simulink model "CubeX_LQR_3D"  (R2017b)
settings: Solver=FixedStepDiscrete  StartTime=0.0  StopTime=inf  FixedStep=Ts.base  RelTol=1e-3
PreLoadFcn:
  | waijung.modelPreload; % Required for working with Waijung Blockset. Do not remove.
InitFcn:
  | cubeparameters
  | LQR_3d
undefined symbols (not defined in the file or in its folder): deg_, g, HSEOSC, imu, K_lqr_3D, Link, LQFP176, motor, ST, STM32F417IG, Ts
libraries: simulink x29, stm32f4_i2c_lib x8, stm32f4_io_lib x7, stm32f4_adc_lib x3, stm32f4_device_config_lib x1, BC_USB x1
(part 1 of 3)
CloseFcn:
  | waijung.modelClose; % Required for working with Waijung Blockset. Do not remove.
settings Model: Creator=Hi  LastModifiedBy=Love
settings DataIOCC: LimitDataPoints=on  SaveFormat=Array
settings OptimizationCC: LifeSpan=1
settings DebuggingCC: AllowSymbolicDim=off  SFUnexpectedBacktrackingDiag=warning  SFNoUnconditionalDefaultTransitionDiag=warning  SFExecutionAtInitializationDiag=none
settings HardwareCC: ProdBitPerPointer=32  ProdBitPerSizeT=32  ProdBitPerPtrDiffT=32  ProdLargestAtomicFloat=None  ProdIntDivRoundTo=Undefined  ProdWordSize=32  ProdHWDeviceType=ARM Compatible->Cortex - M4  TargetEndianess=LittleEndian  TargetHWDeviceType=ARM Compatible->Cortex - M4
settings ModelReferenceCC: PropagateSignalLabelsOutOfModel=off
settings SFSimCC: MATLABDynamicMemAlloc=off
settings RTWCC: SystemTargetFile=stm32f4.tlc  GenerateMakefile=off  TemplateMakefile=ert_default_tmf  Description=STM32F4 Target
settings CodeAppCC: ForceParamTrailComments=on  IgnoreCustomStorageClasses=off  OperatorAnnotations=on  SimulinkDataObjDesc=on  InsertBlockDesc=on  StateflowObjectComments=on  MATLABSourceComments=on
settings STFCustomTargetCC: ModelReferenceCompliant=off  CombineOutputUpdateFcns=on  ERTCustomFileBanners=on  SupportContinuousTime=off  SupportNonInlinedSFcns=off  RemoveResetFunc=on  MATLABClassNameForMDSCustomization=Simulink.SoftwareTarget.ERTCustomization  GRTInterface=off  SystemTargetFile=stm32f4.tlc
settings ERTTargetCC: MultiwordLength=2048  ModelReferenceCompliant=off  ParMdlRefBuildCompliant=off  CompOptLevelCompliant=off  ConcurrentExecutionCompliant=off  ModelStepFunctionPrototypeControlCompliant=off  CPPClassGenCompliant=off  UseToolchainInfoCompliant=off  ERTSrcFileBannerTemplate=stm32f4_code_template.cgt  ERTHdrFileBannerTemplate=stm32f4_code_template.cgt  ERTDataSrcFileTemplate=stm32f4_code_template.cgt  ERTDataHdrFileTemplate=stm32f4_code_template.cgt  ERTCustomFileTemplate=stm32f4_file_process.tlc  ConvertIfToSwitch=off  SuppressUnreachableDefaultCases=off
settings ConfigComp: CovMetricSettings=dw  CovHtmlReporting=on  CovSaveCumulativeToWorkspaceVar=on  CovSaveSingleToWorkspaceVar=on  CovExternalEMLEnable=off

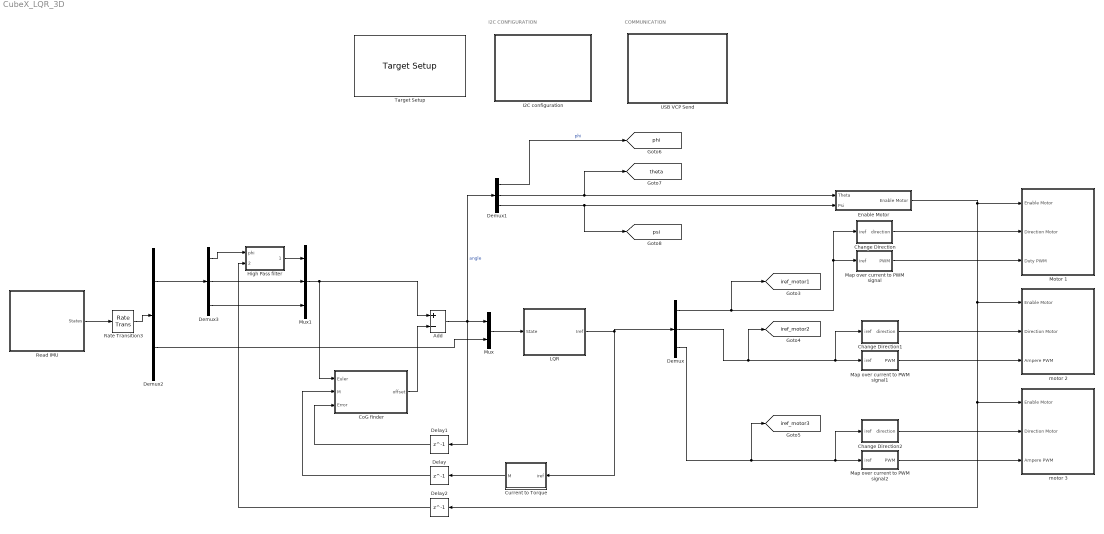
== system CubeX_LQR_3D ==
  note: COMMUNICATION
  note: I2C CONFIGURATION
  Add : Sum  Inputs=+-
  Change Direction : Subsystem
  Change Direction1 : Subsystem
  Change Direction2 : Subsystem
  CoG finder : Subsystem
  Current to Torque : Subsystem
  Delay : Delay  DelayLength=1  InitialCondition=[0 0 0]'
  Delay1 : Delay  DelayLength=1  InitialCondition=[0 0 0]'
  Delay2 : Delay  DelayLength=1  InitialCondition=0
  Demux : Demux  Outputs=3
  Demux1 : Demux  Outputs=3
  Demux2 : Demux  Outputs=2
  Demux3 : Demux  Outputs=3
  Enable Motor : Subsystem  SystemSampleTime=Ts.controller
  High Pass filter : MATLAB Function  TreatAsAtomicUnit=on
  I2C configuration : Subsystem
  LQR : Subsystem
  Map over current to PWM signal : Subsystem
  Map over current to PWM signal1 : Subsystem
  Map over current to PWM signal2 : Subsystem
  Motor 1 : Subsystem
  Mux : Mux  Inputs=2
  Mux1 : Mux  Inputs=3
  Rate Transition3 : RateTransition  OutPortSampleTime=Ts.controller
  Read IMU : Subsystem
  Target Setup : stm32f4_device_config_lib/Target Setup  Priority=100  compiler=GNU ARM  previous_compiler=GNU ARM  mcu=STM32F417IG (LQFP176)  mcustr=STM32F417IG  clockconfig=HSEOSC-8MHz  system_stm32f4xx_c_path=C:\waijung15_04a\targets\stm32f4_target\stm32f4\utils\STM32F4xx_AN3988_V1.0.1\stm32f4_default\hseosc8mhz  showmemoryconfiguration=off  stacksize=0x400  heapsize=0x200  enableautocompiledownload=on  fullchiperase=off  programmerinterface=ST-Link  editctrlstr=on  compilercontrolstr=$(patsubst %, -I%, .) -mcpu=cortex-m4 -mthumb -mthumb-interwork -mfloat-abi=hard -mfpu=fpv4-sp-d16 -ffast-math -Wall -Wextra -Ofast  assemblercontrolstr=$(patsubst %, -I%, .) -mcpu=cortex-m4 -mthumb -mthumb-interwork -mfloat-abi=hard -mfpu=fpv4-sp-d16 -ffast-math -Wall -Wextra -Ofast -Wa,-amhls=$(<:.s=.lst) -D__STACK_SIZE=$(STACK_SIZE) -D__HEAP_SIZE=$(HEAP_SIZE)  linkercontrolstr=-T$(LD_SCRIPT) -g -Wl,-Map=$(MAP),--cref,--no-warn-mismatch -mcpu=cortex-m4 -mthumb -mthumb-interwork -mfloat-abi=hard -mfpu=fpv4-sp-d16  runafterdownload=on  execprofile=None  profileruart=1  profilerbaud=115200  profilertxpin=D8  profilerinitstr=0.002,168000000,336000,115200,0  manualsetsampletime=on  sampletime=0.002  blockid=TargetSetup  systickreloadvalue=336000  hseval=8000000  lastprofileruart=1  hclk=168000000  flashorigin=0x8000000  flashlength=1M  ramorigin=0x20000000  ramlength=112k  useextram=off
  USB VCP Send : Subsystem
  motor 2 : Subsystem
  "motor 3 " : Subsystem
  tag scope: iref_motor1=global, iref_motor2=global, iref_motor3=global, phi=global, psi=global, theta=global
  wires:
  Map over current to PWM signal/1(PWM) -> Motor 1/3(Duty PWM)
  Change Direction/1(direction) -> Motor 1/2("Direction Motor ")
  Enable Motor/1(Enable Motor) -> motor 2/1(Enable Motor), "motor 3 "/1(Enable Motor), Delay2/1, Motor 1/1(Enable Motor)
  CoG finder/1(offset) -> Add/2
  Change Direction1/1(direction) -> motor 2/2("Direction Motor ")
  Change Direction2/1(direction) -> "motor 3 "/2("Direction Motor ")
  Map over current to PWM signal2/1(PWM) -> "motor 3 "/3(Ampere PWM)
  Map over current to PWM signal1/1(PWM) -> motor 2/3(Ampere PWM)
  Add/1 -> Demux1/1, Delay1/1, Mux/1  "angle"
  Mux/1 -> LQR/1(State)
  LQR/1(Iref) -> Current to Torque/1(iref), Demux/1
  Read IMU/1(States) -> Rate Transition3/1
  Rate Transition3/1 -> Demux2/1
  Demux2/2 -> Mux/2
  Delay/1 -> CoG finder/2(M)
  Delay1/1 -> CoG finder/3(Error)
  Demux2/1 -> Demux3/1
  Demux3/1 -> High Pass filter/1(phi)
  High Pass filter/1(phi_zero) -> Mux1/1
  Demux3/2 -> Mux1/2
  Demux3/3 -> Mux1/3
  Mux1/1 -> CoG finder/1(Euler), Add/1
  Delay2/1 -> High Pass filter/2(motor_enable)
  Demux1/2 -> [theta], Enable Motor/1(Theta)
  Demux1/3 -> [psi], Enable Motor/2(Psi)
  Demux1/1 -> [phi]  "phi"
  Demux/2 -> Change Direction1/1(iref), Map over current to PWM signal1/1(iref), [iref_motor2]
  Demux/3 -> Change Direction2/1(iref), Map over current to PWM signal2/1(iref), [iref_motor3]
  Demux/1 -> [iref_motor1], Change Direction/1(iref), Map over current to PWM signal/1(iref)
  Current to Torque/1(M) -> Delay/1

== system CubeX_LQR_3D/Change Direction ==
  iref : Inport
  Compare To Zero : simulink/Logic and Bit Operations/Compare To Zero  relop=>=  OutDataTypeStr=boolean
  direction : Outport
  wires:
  iref/1 -> Compare To Zero/1
  Compare To Zero/1 -> direction/1

== system CubeX_LQR_3D/Change Direction1 ==
  iref : Inport
  Compare To Zero : simulink/Logic and Bit Operations/Compare To Zero  relop=>=  OutDataTypeStr=boolean
  direction : Outport
  wires:
  iref/1 -> Compare To Zero/1
  Compare To Zero/1 -> direction/1

== system CubeX_LQR_3D/Change Direction2 ==
  iref : Inport
  Compare To Zero : simulink/Logic and Bit Operations/Compare To Zero  relop=>=  OutDataTypeStr=boolean
  direction : Outport
  wires:
  iref/1 -> Compare To Zero/1
  Compare To Zero/1 -> direction/1

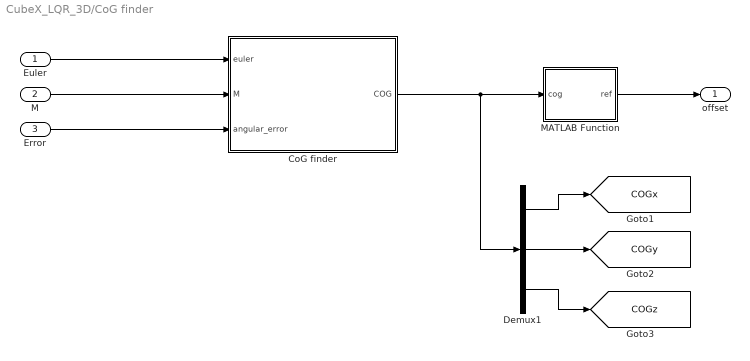
== system CubeX_LQR_3D/CoG finder ==
  Euler : Inport
  M : Inport  Port=2
  Error : Inport  Port=3
  CoG finder : MATLAB Function  TreatAsAtomicUnit=on
  Demux1 : Demux  Outputs=3
  MATLAB Function : MATLAB Function  TreatAsAtomicUnit=on
  offset : Outport
  tag scope: COGx=global, COGy=global, COGz=global
  wires:
  CoG finder/1(COG) -> Demux1/1, MATLAB Function/1(cog)
  MATLAB Function/1(ref) -> offset/1
  Demux1/2 -> [COGy]
  Demux1/3 -> [COGz]
  Demux1/1 -> [COGx]
  Euler/1 -> CoG finder/1(euler)
  Error/1 -> CoG finder/3(angular_error)
  M/1 -> CoG finder/2(M)

== system CubeX_LQR_3D/Current to Torque ==
  iref : Inport
  "Gain " : Gain  Gain=motor.kt
  M : Outport
  wires:
  iref/1 -> "Gain "/1
  "Gain "/1 -> M/1

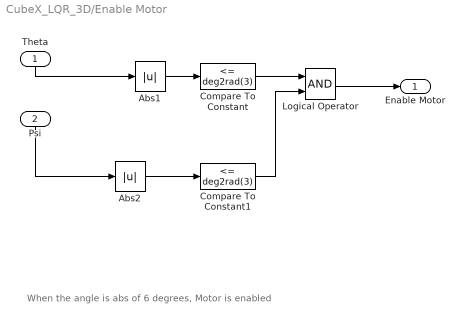
== system CubeX_LQR_3D/Enable Motor ==
  note: When the angle is abs of 6 degrees, Motor is enabled
  Theta : Inport
  Psi : Inport  Port=2
  Abs1 : Abs
  Abs2 : Abs
  Compare To Constant : simulink/Logic and Bit Operations/Compare To Constant  relop=<=  const=deg2rad(3)  OutDataTypeStr=boolean
  Compare To Constant1 : simulink/Logic and Bit Operations/Compare To Constant  relop=<=  const=deg2rad(3)  OutDataTypeStr=boolean
  Logical Operator : Logic  AllPortsSameDT=off  OutDataTypeStr=boolean
  Enable Motor : Outport
  wires:
  Abs1/1 -> Compare To Constant/1
  Theta/1 -> Abs1/1
  Psi/1 -> Abs2/1
  Abs2/1 -> Compare To Constant1/1
  Compare To Constant/1 -> Logical Operator/1
  Compare To Constant1/1 -> Logical Operator/2
  Logical Operator/1 -> Enable Motor/1

== system CubeX_LQR_3D/I2C configuration ==
  I2C Master Setup1 : S-Function  FunctionName=stm32f4_i2c  Parameters=configuration,module,transfer,clkspeed,timeout,sdapin,sclpin,writecount,readcount,inputtypearray,outputtypearray,confstr,sampletime,sampletimestr,blockid  SFunctionDeploymentMode=off  EnableBusSupport=off  mask(stm32f4_i2c){configuration=Setup, module=3, lastmodule=3, transfer=Blocking, dutycycle=TLow/THigh = 2, clkspeed=400, timeout=25, writecount=0, readcount=0, sdapin=C9, sclpin=A8, waitwritetime=0, inputtypearray=[0], outputtypearray=[0], confstr=["C","9","A","8","1","3","4","2","I2C_DutyCycle_2","0","off"], sampletime=-1, sampletimestr=0.002, blockid=I2CconfigurationI2CMasterSetup1}
      mask prompts: module "I2C Module"; lastmodule "Last module"; transfer "Transfer mode"; dutycycle "Duty cycle in fast mode"; clkspeed "Clock speed (kHz)"; timeout "Timeout (ms)"; writecount "Bytes write count"; readcount "Bytes read count"; sdapin "SDA pin"; sclpin "SCL pin"; waitwritetime "Wait write time (ms), default is 0"; inputtypearray "Input type array"; outputtypearray "Output type array"; confstr "Configuration string"; sampletime "Sample time (sec)"; sampletimestr "Compiled sample time (sec) in string"
      mask init:
      | stm32f4_i2c_callback('init');
      mask Help: web(fullfile(waijungdocroot,'stm32f4_i2c_setup.htm'), '-browser')
      mask TypeOptions configuration: Setup | Transaction
      mask Callback configuration: stm32f4_i2c_callback('configuration');
      mask TypeOptions module: 1 | 2 | 3
      mask Callback module: stm32f4_i2c_callback('module');
      mask TypeOptions transfer: Blocking | Non-blocking
      mask TypeOptions dutycycle: TLow/THigh = 16/9 | TLow/THigh = 2
      mask Callback dutycycle: stm32f4_i2c_callback('dutycycle');
      mask Callback writecount: stm32f4_i2c_callback('writecount');
      mask Callback readcount: stm32f4_i2c_callback('readcount');
      mask TypeOptions sdapin: - | C9
      mask Callback sdapin: stm32f4_i2c_callback('sdapin');
      mask TypeOptions sclpin: - | A8
      mask Callback sclpin: stm32f4_i2c_callback('sclpin');
      mask Callback confstr: stm32f4_i2c_callback('confstr');
      mask Callback sampletime: stm32f4_i2c_callback('sampletime');
      mask Callback sampletimestr: stm32f4_i2c_callback('sampletimestr');
      mask Callback blockid: stm32f4_i2c_callback('blockid');
      mask Display: text(0.5, 0.5, 'Module: I2C3\nClock: 400kHz\nSDA/SCL Pin: C9/A8','ver','middle','hor','center');
  I2C Master Setup2 : S-Function  FunctionName=stm32f4_i2c  Parameters=configuration,module,transfer,clkspeed,timeout,sdapin,sclpin,writecount,readcount,inputtypearray,outputtypearray,confstr,sampletime,sampletimestr,blockid  SFunctionDeploymentMode=off  EnableBusSupport=off  mask(stm32f4_i2c){configuration=Setup, module=1, lastmodule=1, transfer=Blocking, dutycycle=TLow/THigh = 2, clkspeed=400, timeout=25, writecount=0, readcount=0, sdapin=B9, sclpin=B6, waitwritetime=0, inputtypearray=[0], outputtypearray=[0], confstr=["B","9","B","6","1","1","6","0","I2C_DutyCycle_2","0","off"], sampletime=-1, sampletimestr=0.002, blockid=I2CconfigurationI2CMasterSetup2}
      mask prompts: module "I2C Module"; lastmodule "Last module"; transfer "Transfer mode"; dutycycle "Duty cycle in fast mode"; clkspeed "Clock speed (kHz)"; timeout "Timeout (ms)"; writecount "Bytes write count"; readcount "Bytes read count"; sdapin "SDA pin"; sclpin "SCL pin"; waitwritetime "Wait write time (ms), default is 0"; inputtypearray "Input type array"; outputtypearray "Output type array"; confstr "Configuration string"; sampletime "Sample time (sec)"; sampletimestr "Compiled sample time (sec) in string"
      mask init:
      | stm32f4_i2c_callback('init');
      mask Help: web(fullfile(waijungdocroot,'stm32f4_i2c_setup.htm'), '-browser')
      mask TypeOptions configuration: Setup | Transaction
      mask Callback configuration: stm32f4_i2c_callback('configuration');
      mask TypeOptions module: 1 | 2 | 3
      mask Callback module: stm32f4_i2c_callback('module');
      mask TypeOptions transfer: Blocking | Non-blocking
      mask TypeOptions dutycycle: TLow/THigh = 16/9 | TLow/THigh = 2
      mask Callback dutycycle: stm32f4_i2c_callback('dutycycle');
      mask Callback writecount: stm32f4_i2c_callback('writecount');
      mask Callback readcount: stm32f4_i2c_callback('readcount');
      mask TypeOptions sdapin: - | B7 | B9
      mask Callback sdapin: stm32f4_i2c_callback('sdapin');
      mask TypeOptions sclpin: - | B6 | B8
      mask Callback sclpin: stm32f4_i2c_callback('sclpin');
      mask Callback confstr: stm32f4_i2c_callback('confstr');
      mask Callback sampletime: stm32f4_i2c_callback('sampletime');
      mask Callback sampletimestr: stm32f4_i2c_callback('sampletimestr');
      mask Callback blockid: stm32f4_i2c_callback('blockid');
      mask Display: text(0.5, 0.5, 'Module: I2C1\nClock: 400kHz\nSDA/SCL Pin: B9/B6','ver','middle','hor','center');

== system CubeX_LQR_3D/LQR ==
  State : Inport
  K matrix (LQR) : Subsystem
  Torque to Current : Subsystem
  Iref : Outport
  wires:
  Torque to Current/1(iref) -> Iref/1
  State/1 -> K matrix (LQR)/1(State)
  K matrix (LQR)/1(M) -> Torque to Current/1(M)

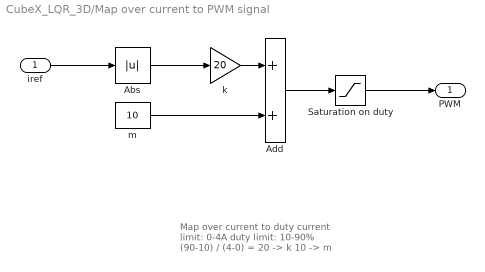
== system CubeX_LQR_3D/Map over current to PWM signal ==
  note: Map over current to duty
      | current limit: 0-4A
      | duty limit: 10-90%
      |
      | (90-10) / (4-0) = 20 -> k
      | 10 -> m
  iref : Inport
  Abs : Abs
  Add : Sum
  Saturation on duty : Saturate  UpperLimit=90  LowerLimit=10  OutDataTypeStr=single
  k : Gain  Gain=20
  m : Constant  Value=10  OutDataTypeStr=single  SampleTime=Ts.controller
  PWM : Outport
  wires:
  Add/1 -> Saturation on duty/1
  Saturation on duty/1 -> PWM/1
  iref/1 -> Abs/1
  Abs/1 -> k/1
  k/1 -> Add/1
  m/1 -> Add/2

== system CubeX_LQR_3D/Map over current to PWM signal1 ==
  note: Map over current to duty
      | current limit: 0-4A
      | duty limit: 10-90%
      |
      | (90-10) / (4-0) = 20 -> k
      | 10 -> m
  iref : Inport
  Abs : Abs
  Add : Sum
  Saturation on duty : Saturate  UpperLimit=90  LowerLimit=10  OutDataTypeStr=single
  k : Gain  Gain=20
  m : Constant  Value=10  OutDataTypeStr=single  SampleTime=Ts.controller
  PWM : Outport
  wires:
  Add/1 -> Saturation on duty/1
  Saturation on duty/1 -> PWM/1
  iref/1 -> Abs/1
  Abs/1 -> k/1
  k/1 -> Add/1
  m/1 -> Add/2

== system CubeX_LQR_3D/Map over current to PWM signal2 ==
  note: Map over current to duty
      | current limit: 0-4A
      | duty limit: 10-90%
      |
      | (90-10) / (4-0) = 20 -> k
      | 10 -> m
  iref : Inport
  Abs : Abs
  Add : Sum
  Saturation on duty : Saturate  UpperLimit=90  LowerLimit=10  OutDataTypeStr=single
  k : Gain  Gain=20
  m : Constant  Value=10  OutDataTypeStr=single  SampleTime=Ts.controller
  PWM : Outport
  wires:
  Add/1 -> Saturation on duty/1
  Saturation on duty/1 -> PWM/1
  iref/1 -> Abs/1
  Abs/1 -> k/1
  k/1 -> Add/1
  m/1 -> Add/2

== system CubeX_LQR_3D/Motor 1 ==
  Enable Motor : Inport
  "Direction Motor " : Inport  Port=2
  Duty PWM : Inport  Port=3
  Direction Motor 1 (green) : stm32f4_io_lib/Digital Output  use_bitband=on  port=D  speed=100  porttype=Push Pull  porttypestr=PP  use_pin0=off  use_pin1=off  use_pin2=off  use_pin3=off  use_pin4=off  use_pin5=off  use_pin6=off  use_pin7=off  use_pin8=off  use_pin9=off  use_pin10=off  use_pin11=on  use_pin12=off  use_pin13=off  use_pin14=off  use_pin15=off  pinstr=GPIO_Pin_11  usedpinarray="[0  0  0  0  0  0  0  0  0  0  0  1  0  0  0  0]"  bitbandingstr="#define Motor1DirectionMotor3green_D11 Peripheral_BB(GPIOD->ODR, 11)  /* Output pin */"  sampletime=-1  sampletimestr=0.016  blockid=Motor1DirectionMotor3green  enablecustomportlabel=off  globalinit=off  cinputportlabel=In1, In2  coutputportlabel=0
  Enable Motor 1(yellow) : stm32f4_io_lib/Digital Output  use_bitband=on  port=D  speed=100  porttype=Push Pull  porttypestr=PP  use_pin0=off  use_pin1=off  use_pin2=off  use_pin3=off  use_pin4=off  use_pin5=off  use_pin6=off  use_pin7=off  use_pin8=off  use_pin9=on  use_pin10=off  use_pin11=off  use_pin12=off  use_pin13=off  use_pin14=off  use_pin15=off  pinstr=GPIO_Pin_9  usedpinarray="[0  0  0  0  0  0  0  0  0  1  0  0  0  0  0  0]"  bitbandingstr="#define Motor1EnableMotor3yellow_D9 Peripheral_BB(GPIOD->ODR, 9)  /* Output pin */"  sampletime=-1  sampletimestr=-1  blockid=Motor1EnableMotor3yellow  enablecustomportlabel=off  globalinit=off  cinputportlabel=In1, In2  coutputportlabel=0
  PWM Ampere motor 1 (white) : S-Function  FunctionName=stm32f4_basicpwm_fixed  Parameters=timer,pwmperiod,uc3m_pwmperiod,ch1pin,ch2pin,ch3pin,ch4pin,sampletime,sampletimestr,blockid,apb,portstr,pinstr,pinmat,timarr,timprescale,chmat,polaritystr  SFunctionDeploymentMode=off  EnableBusSupport=off  mask(stm32f4_basicpwm_fixed){timer=2, pwmperiod=0.02, uc3m_pwmperiod=0.0002, polarity=Active High, polaritystr=TIM_OCPolarity_High, ch1pin=Not available - Do not use, ch2pin=Not available - Do not use, ch3pin=Not available - Do not use, ch4pin=A3, sampletime=-1, sampletimestr=0.016, blockid=Motor1PWMAmperemotor3, portpinstr=,,,A3, enablecustomportlabel=off, cinputportlabel=In1, In2, In3, In4, coutputportlabel=0, callbackgensrccode=off, apb=1, portstr=["A"], pinstr=["GPIO_Pin_3"], pinmat=[1 3], timarr=59999, timprescale=55, chmat=[4]}
      mask prompts: pwmperiod "PWM Period (seconds)"; uc3m_pwmperiod "PWM Signal Period (seconds)"; ch1pin "Channel 1"; ch2pin "Channel 2"; ch3pin "Channel 3"; ch4pin "Channel 4"; sampletime "Sample time (sec)"; sampletimestr "Compiled sample time (sec) in string"; portpinstr "Port pin string"; enablecustomportlabel "Enable custom port labels"; cinputportlabel "Custom input port labels (Ex. In1, In2, In3)"; coutputportlabel "Custom output port labels (Ex. Out1, Out2, Out3)"; callbackgensrccode "Gen source code from callback"; portstr "Port string"; pinstr "Pin string"; pinmat "Pin matrix"; timarr "Timer ARR"; timprescale "Timer PRESCALE"; chmat "Channel order"
      mask help:
      | This block implements basic Edge-aligned Pulse Width Modulation (PWM) generation.
      | All timers are 16-bit. The PWM period is fixed (per timer).
      |
      | This block was fixed by Sr Antonio
      mask init:
      | stm32f4_basicpwm_callback_fixed('init');
      mask Help: web(fullfile(waijungdocroot,'stm32f4_basicpwm.htm'),'-browser')
      mask TypeOptions timer: 1 | 2 | 3 | 4 | 5 | 8 | 9 | 10 | 11 | 12 | 13 | 14
      mask Callback timer: stm32f4_basicpwm_callback_fixed('timer');
      mask Callback pwmperiod: stm32f4_basicpwm_callback_fixed('pwmperiod');
      mask Callback uc3m_pwmperiod: stm32f4_basicpwm_callback_fixed('uc3m_pwmperiod');
      mask TypeOptions polarity: Active High | Active Low
      mask Callback polarity: stm32f4_basicpwm_callback_fixed('polarity');
      mask TypeOptions ch1pin: Not available - Do not use | A0 | A5
      mask Callback ch1pin: stm32f4_basicpwm_callback_fixed('ch1pin');
      mask TypeOptions ch2pin: Not available - Do not use | A1 | B3
      mask Callback ch2pin: stm32f4_basicpwm_callback_fixed('ch2pin');
      mask TypeOptions ch3pin: Not available - Do not use | A2 | B10
      mask Callback ch3pin: stm32f4_basicpwm_callback_fixed('ch3pin');
      mask TypeOptions ch4pin: Not available - Do not use | A3 | B11
      mask Callback ch4pin: stm32f4_basicpwm_callback_fixed('ch4pin');
      mask Callback sampletime: stm32f4_basicpwm_callback_fixed('sampletime');
      mask Callback sampletimestr: stm32f4_basicpwm_callback_fixed('sampletimestr');
      mask Callback blockid: stm32f4_basicpwm_callback_fixed('blockid');
      mask Callback enablecustomportlabel: stm32f4_basicpwm_callback_fixed('enablecustomportlabel')
      mask Display: text(0.95, 0.5, 'UC3M FIXED\nTimer: 2\nPolarity: Active High\nPeriod (sec): 0.0002\nTs (sec): -1','ver','middle','hor','right');port_label('input', 1,'CH4 (A3)')
  "Velocty wheel 3, analog in (Grey), PC1" : stm32f4_adc_lib/Regular ADC  Commented=on  adcmodule=3  outputdatatype=Single  prescaler=2  prescalerstr=ADC_Prescaler_Div2  chsamplingtime=Auto  chsamplingtimestr=ADC_SampleTime_480Cycles  read_an0=off  read_an1=off  read_an2=off  read_an3=off  read_an4=off  read_an5=off  read_an6=off  read_an7=off  read_an8=off  read_an9=off  read_an10=off  read_an11=on  read_an12=off  read_an13=off  read_an14=off  read_an15=off  read_an16=off  read_an17=off  read_an18=off  pinstr=GPIO_Pin_11  usedpinarray="[0  0  0  0  0  0  0  0  0  0  0  1  0  0  0  0  0  0  0]"  usedportidarray=[2]  usedpinidarray=[1]  usedpinidcount=1  sampletime=Ts.controller  blockid=Motor3Veloctywheel3analoginGreyPC1  enablecustomportlabel=off  cinputportlabel=0  coutputportlabel=Out1, Out2
  wires:
  Duty PWM/1 -> PWM Ampere motor 1 (white)/1
  "Direction Motor "/1 -> Direction Motor 1 (green)/1
  Enable Motor/1 -> Enable Motor 1(yellow)/1

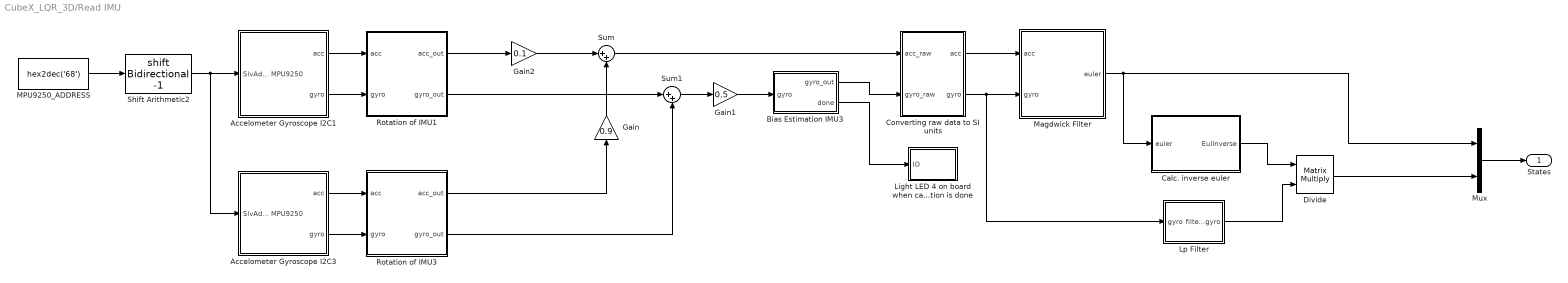
== system CubeX_LQR_3D/Read IMU ==
  " MPU9250_ADDRESS" : Constant  Value=hex2dec('68')  OutDataTypeStr=uint8  SampleTime=Ts.IMU
  Accelometer Gyroscope I2C1 : Subsystem
  Accelometer Gyroscope I2C3 : Subsystem
  Bias Estimation IMU3 : MATLAB Function  TreatAsAtomicUnit=on
  Calc. inverse euler : MATLAB Function  TreatAsAtomicUnit=on
  Converting raw data to SI units : Subsystem
  Divide : Product  Inputs=**  Multiplication=Matrix(*)
  Gain : Gain  Gain=0.9
  Gain1 : Gain  Gain=0.5
  Gain2 : Gain  Gain=0.1
  Light LED 4 on board when calibration is done : Subsystem
  Lp Filter : MATLAB Function  TreatAsAtomicUnit=on
  Magdwick Filter : MATLAB Function  TreatAsAtomicUnit=on
  Mux : Mux  Inputs=2
  Rotation of IMU1 : MATLAB Function  TreatAsAtomicUnit=on
  Rotation of IMU3 : MATLAB Function  TreatAsAtomicUnit=on
  Shift Arithmetic2 : ArithShift  BitShiftNumber=-1
  Sum : Sum  Inputs=|++
  Sum1 : Sum  Inputs=|++
  States : Outport
  wires:
  Converting raw data to SI units/1(acc) -> Magdwick Filter/1(acc)
  Converting raw data to SI units/2(gyro) -> Magdwick Filter/2(gyro), Lp Filter/1(gyro)
  Accelometer Gyroscope I2C1/2(gyro) -> Rotation of IMU1/2(gyro)
  Shift Arithmetic2/1 -> Accelometer Gyroscope I2C3/1(SlvAddr MPU9250), Accelometer Gyroscope I2C1/1(SlvAddr MPU9250)
  Accelometer Gyroscope I2C1/1(acc) -> Rotation of IMU1/1(acc)
  " MPU9250_ADDRESS"/1 -> Shift Arithmetic2/1
  Accelometer Gyroscope I2C3/1(acc) -> Rotation of IMU3/1(acc)
  Accelometer Gyroscope I2C3/2(gyro) -> Rotation of IMU3/2(gyro)
  Sum1/1 -> Gain1/1
  Sum/1 -> Converting raw data to SI units/1(acc_raw)
  Rotation of IMU1/2(gyro_out) -> Sum1/1
  Gain2/1 -> Sum/1
  Gain/1 -> Sum/2
  Gain1/1 -> Bias Estimation IMU3/1(gyro)
  Rotation of IMU3/2(gyro_out) -> Sum1/2
  Rotation of IMU3/1(acc_out) -> Gain/1
  Rotation of IMU1/1(acc_out) -> Gain2/1
  Calc. inverse euler/1(EulInverse) -> Divide/1
  Divide/1 -> Mux/2
  Magdwick Filter/1(euler) -> Mux/1, Calc. inverse euler/1(euler)
  Mux/1 -> States/1
  Lp Filter/1(filter_gyro) -> Divide/2
  Bias Estimation IMU3/1(gyro_out) -> Converting raw data to SI units/2(gyro_raw)
  Bias Estimation IMU3/2(done) -> Light LED 4 on board when calibration is done/1(IO)

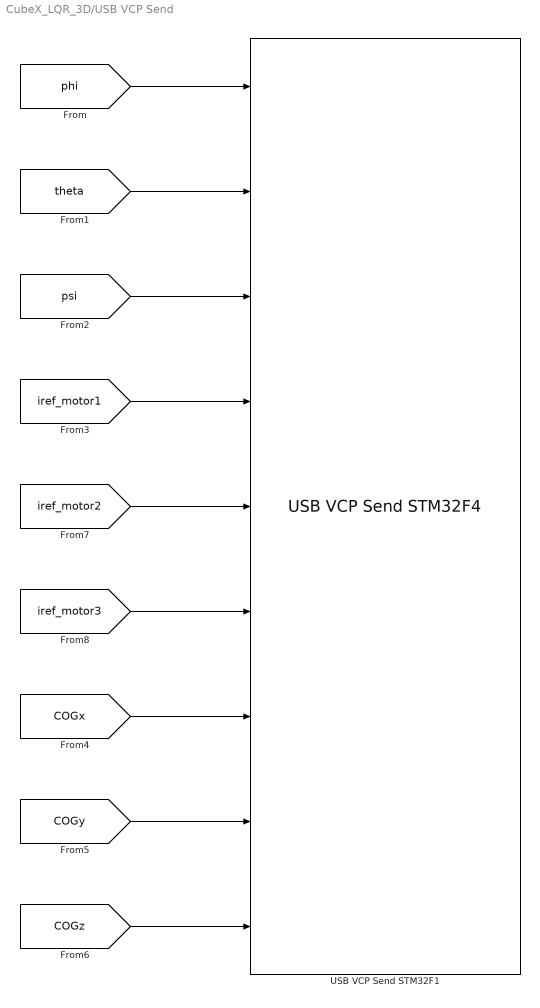
== system CubeX_LQR_3D/USB VCP Send ==
  USB VCP Send STM32F1 : BC_USB/USB VCP Send STM32F4  speed="USB 1.1   12Mbit/s"  data_size=2048 Bytes  header_data='0E 0E'  binary_data='single single single single single single single single single'  terminator_data='0A 0A'  sampletime=Ts.base
  wires:
  [phi] -> USB VCP Send STM32F1/1
  [theta] -> USB VCP Send STM32F1/2
  [psi] -> USB VCP Send STM32F1/3
  [COGx] -> USB VCP Send STM32F1/7
  [COGy] -> USB VCP Send STM32F1/8
  [COGz] -> USB VCP Send STM32F1/9
  [iref_motor1] -> USB VCP Send STM32F1/4
  [iref_motor2] -> USB VCP Send STM32F1/5
  [iref_motor3] -> USB VCP Send STM32F1/6

== system CubeX_LQR_3D/motor 2 ==
  Enable Motor : Inport
  "Direction Motor " : Inport  Port=2
  Ampere PWM : Inport  Port=3
  Direction Motor 2 (green) : stm32f4_io_lib/Digital Output  use_bitband=on  port=E  speed=100  porttype=Push Pull  porttypestr=PP  use_pin0=off  use_pin1=off  use_pin2=off  use_pin3=off  use_pin4=off  use_pin5=off  use_pin6=off  use_pin7=off  use_pin8=on  use_pin9=off  use_pin10=off  use_pin11=off  use_pin12=off  use_pin13=off  use_pin14=off  use_pin15=off  pinstr=GPIO_Pin_8  usedpinarray="[0  0  0  0  0  0  0  0  1  0  0  0  0  0  0  0]"  bitbandingstr="#define motor2DirectionMotor2green_E8 Peripheral_BB(GPIOE->ODR, 8)  /* Output pin */"  sampletime=-1  sampletimestr=0.016  blockid=motor2DirectionMotor2green  enablecustomportlabel=off  globalinit=off  cinputportlabel=In1, In2  coutputportlabel=0
  Enable Motor 2(yellow) : stm32f4_io_lib/Digital Output  use_bitband=on  port=E  speed=100  porttype=Push Pull  porttypestr=PP  use_pin0=off  use_pin1=off  use_pin2=off  use_pin3=off  use_pin4=off  use_pin5=off  use_pin6=off  use_pin7=on  use_pin8=off  use_pin9=off  use_pin10=off  use_pin11=off  use_pin12=off  use_pin13=off  use_pin14=off  use_pin15=off  pinstr=GPIO_Pin_7  usedpinarray="[0  0  0  0  0  0  0  1  0  0  0  0  0  0  0  0]"  bitbandingstr="#define motor2EnableMotor2yellow_E7 Peripheral_BB(GPIOE->ODR, 7)  /* Output pin */"  sampletime=-1  sampletimestr=0.016  blockid=motor2EnableMotor2yellow  enablecustomportlabel=off  globalinit=off  cinputportlabel=In1, In2  coutputportlabel=0
  PWM Ampere motor 2 (white) : S-Function  FunctionName=stm32f4_basicpwm_fixed  Parameters=timer,pwmperiod,uc3m_pwmperiod,ch1pin,ch2pin,ch3pin,ch4pin,sampletime,sampletimestr,blockid,apb,portstr,pinstr,pinmat,timarr,timprescale,chmat,polaritystr  SFunctionDeploymentMode=off  EnableBusSupport=off  mask(stm32f4_basicpwm_fixed){timer=2, pwmperiod=0.02, uc3m_pwmperiod=0.0002, polarity=Active High, polaritystr=TIM_OCPolarity_High, ch1pin=Not available - Do not use, ch2pin=A1, ch3pin=Not available - Do not use, ch4pin=Not available - Do not use, sampletime=-1, sampletimestr=0.016, blockid=motor2PWMAmperemotor2, portpinstr=,A1,,, enablecustomportlabel=off, cinputportlabel=In1, In2, In3, In4, coutputportlabel=0, callbackgensrccode=off, apb=1, portstr=["A"], pinstr=["GPIO_Pin_1"], pinmat=[1 1], timarr=59999, timprescale=55, chmat=[2]}
      mask prompts: pwmperiod "PWM Period (seconds)"; uc3m_pwmperiod "PWM Signal Period (seconds)"; ch1pin "Channel 1"; ch2pin "Channel 2"; ch3pin "Channel 3"; ch4pin "Channel 4"; sampletime "Sample time (sec)"; sampletimestr "Compiled sample time (sec) in string"; portpinstr "Port pin string"; enablecustomportlabel "Enable custom port labels"; cinputportlabel "Custom input port labels (Ex. In1, In2, In3)"; coutputportlabel "Custom output port labels (Ex. Out1, Out2, Out3)"; callbackgensrccode "Gen source code from callback"; portstr "Port string"; pinstr "Pin string"; pinmat "Pin matrix"; timarr "Timer ARR"; timprescale "Timer PRESCALE"; chmat "Channel order"
      mask help:
      | This block implements basic Edge-aligned Pulse Width Modulation (PWM) generation.
      | All timers are 16-bit. The PWM period is fixed (per timer).
      |
      | This block was fixed by Sr Antonio
      mask init:
      | stm32f4_basicpwm_callback_fixed('init');
      mask Help: web(fullfile(waijungdocroot,'stm32f4_basicpwm.htm'),'-browser')
      mask TypeOptions timer: 1 | 2 | 3 | 4 | 5 | 8 | 9 | 10 | 11 | 12 | 13 | 14
      mask Callback timer: stm32f4_basicpwm_callback_fixed('timer');
      mask Callback pwmperiod: stm32f4_basicpwm_callback_fixed('pwmperiod');
      mask Callback uc3m_pwmperiod: stm32f4_basicpwm_callback_fixed('uc3m_pwmperiod');
      mask TypeOptions polarity: Active High | Active Low
      mask Callback polarity: stm32f4_basicpwm_callback_fixed('polarity');
      mask TypeOptions ch1pin: Not available - Do not use | A0 | A5
      mask Callback ch1pin: stm32f4_basicpwm_callback_fixed('ch1pin');
      mask TypeOptions ch2pin: Not available - Do not use | A1 | B3
      mask Callback ch2pin: stm32f4_basicpwm_callback_fixed('ch2pin');
      mask TypeOptions ch3pin: Not available - Do not use | A2 | B10
      mask Callback ch3pin: stm32f4_basicpwm_callback_fixed('ch3pin');
      mask TypeOptions ch4pin: Not available - Do not use | A3 | B11
      mask Callback ch4pin: stm32f4_basicpwm_callback_fixed('ch4pin');
      mask Callback sampletime: stm32f4_basicpwm_callback_fixed('sampletime');
      mask Callback sampletimestr: stm32f4_basicpwm_callback_fixed('sampletimestr');
      mask Callback blockid: stm32f4_basicpwm_callback_fixed('blockid');
      mask Callback enablecustomportlabel: stm32f4_basicpwm_callback_fixed('enablecustomportlabel')
      mask Display: text(0.95, 0.5, 'UC3M FIXED\nTimer: 2\nPolarity: Active High\nPeriod (sec): 0.0002\nTs (sec): -1','ver','middle','hor','right');port_label('input', 1,'CH2 (A1)')
  "Velocty wheel 2, analog in (Grey), PB1" : stm32f4_adc_lib/Regular ADC  Commented=on  adcmodule=2  outputdatatype=Double  prescaler=2  prescalerstr=ADC_Prescaler_Div2  chsamplingtime=Auto  chsamplingtimestr=ADC_SampleTime_480Cycles  read_an0=off  read_an1=off  read_an2=off  read_an3=off  read_an4=off  read_an5=off  read_an6=off  read_an7=off  read_an8=off  read_an9=on  read_an10=off  read_an11=off  read_an12=off  read_an13=off  read_an14=off  read_an15=off  read_an16=off  read_an17=off  read_an18=off  pinstr=GPIO_Pin_9  usedpinarray="[0  0  0  0  0  0  0  0  0  1  0  0  0  0  0  0  0  0  0]"  usedportidarray=[1]  usedpinidarray=[1]  usedpinidcount=1  sampletime=Ts.controller  blockid=motor2Veloctywheel2analoginGreyPB1  enablecustomportlabel=off  cinputportlabel=0  coutputportlabel=Out1, Out2
  wires:
  Enable Motor/1 -> Enable Motor 2(yellow)/1
  Ampere PWM/1 -> PWM Ampere motor 2 (white)/1
  "Direction Motor "/1 -> Direction Motor 2 (green)/1

== system CubeX_LQR_3D/motor 3  ==
  Enable Motor : Inport
  "Direction Motor " : Inport  Port=2
  Ampere PWM : Inport  Port=3
  Direction Motor 3 (green) : stm32f4_io_lib/Digital Output  use_bitband=on  port=B  speed=100  porttype=Push Pull  porttypestr=PP  use_pin0=off  use_pin1=off  use_pin2=on  use_pin3=off  use_pin4=off  use_pin5=off  use_pin6=off  use_pin7=off  use_pin8=off  use_pin9=off  use_pin10=off  use_pin11=off  use_pin12=off  use_pin13=off  use_pin14=off  use_pin15=off  pinstr=GPIO_Pin_2  usedpinarray="[0  0  1  0  0  0  0  0  0  0  0  0  0  0  0  0]"  bitbandingstr="#define motor3DirectionMotor3green_B2 Peripheral_BB(GPIOB->ODR, 2)  /* Output pin */"  sampletime=-1  sampletimestr=0.016  blockid=motor3DirectionMotor3green  enablecustomportlabel=off  globalinit=off  cinputportlabel=In1, In2  coutputportlabel=0
  Enable Motor 3(yellow) : stm32f4_io_lib/Digital Output  use_bitband=on  port=B  speed=100  porttype=Push Pull  porttypestr=PP  use_pin0=on  use_pin1=off  use_pin2=off  use_pin3=off  use_pin4=off  use_pin5=off  use_pin6=off  use_pin7=off  use_pin8=off  use_pin9=off  use_pin10=off  use_pin11=off  use_pin12=off  use_pin13=off  use_pin14=off  use_pin15=off  pinstr=GPIO_Pin_0  usedpinarray="[1  0  0  0  0  0  0  0  0  0  0  0  0  0  0  0]"  bitbandingstr="#define motor3EnableMotor3yellow_B0 Peripheral_BB(GPIOB->ODR, 0)  /* Output pin */"  sampletime=-1  sampletimestr=0.016  blockid=motor3EnableMotor3yellow  enablecustomportlabel=off  globalinit=off  cinputportlabel=In1, In2  coutputportlabel=0
  PWM Ampere motor 3 (white) : S-Function  FunctionName=stm32f4_basicpwm_fixed  Parameters=timer,pwmperiod,uc3m_pwmperiod,ch1pin,ch2pin,ch3pin,ch4pin,sampletime,sampletimestr,blockid,apb,portstr,pinstr,pinmat,timarr,timprescale,chmat,polaritystr  SFunctionDeploymentMode=off  EnableBusSupport=off  mask(stm32f4_basicpwm_fixed){timer=2, pwmperiod=0.02, uc3m_pwmperiod=0.0002, polarity=Active High, polaritystr=TIM_OCPolarity_High, ch1pin=Not available - Do not use, ch2pin=Not available - Do not use, ch3pin=A2, ch4pin=Not available - Do not use, sampletime=-1, sampletimestr=0.016, blockid=motor3PWMAmperemotor3, portpinstr=,,A2,, enablecustomportlabel=off, cinputportlabel=In1, In2, In3, In4, coutputportlabel=0, callbackgensrccode=off, apb=1, portstr=["A"], pinstr=["GPIO_Pin_2"], pinmat=[1 2], timarr=59999, timprescale=55, chmat=[3]}
      mask prompts: pwmperiod "PWM Period (seconds)"; uc3m_pwmperiod "PWM Signal Period (seconds)"; ch1pin "Channel 1"; ch2pin "Channel 2"; ch3pin "Channel 3"; ch4pin "Channel 4"; sampletime "Sample time (sec)"; sampletimestr "Compiled sample time (sec) in string"; portpinstr "Port pin string"; enablecustomportlabel "Enable custom port labels"; cinputportlabel "Custom input port labels (Ex. In1, In2, In3)"; coutputportlabel "Custom output port labels (Ex. Out1, Out2, Out3)"; callbackgensrccode "Gen source code from callback"; portstr "Port string"; pinstr "Pin string"; pinmat "Pin matrix"; timarr "Timer ARR"; timprescale "Timer PRESCALE"; chmat "Channel order"
      mask help:
      | This block implements basic Edge-aligned Pulse Width Modulation (PWM) generation.
      | All timers are 16-bit. The PWM period is fixed (per timer).
      |
      | This block was fixed by Sr Antonio
      mask init:
      | stm32f4_basicpwm_callback_fixed('init');
      mask Help: web(fullfile(waijungdocroot,'stm32f4_basicpwm.htm'),'-browser')
      mask TypeOptions timer: 1 | 2 | 3 | 4 | 5 | 8 | 9 | 10 | 11 | 12 | 13 | 14
      mask Callback timer: stm32f4_basicpwm_callback_fixed('timer');
      mask Callback pwmperiod: stm32f4_basicpwm_callback_fixed('pwmperiod');
      mask Callback uc3m_pwmperiod: stm32f4_basicpwm_callback_fixed('uc3m_pwmperiod');
      mask TypeOptions polarity: Active High | Active Low
      mask Callback polarity: stm32f4_basicpwm_callback_fixed('polarity');
      mask TypeOptions ch1pin: Not available - Do not use | A0 | A5
      mask Callback ch1pin: stm32f4_basicpwm_callback_fixed('ch1pin');
      mask TypeOptions ch2pin: Not available - Do not use | A1 | B3
      mask Callback ch2pin: stm32f4_basicpwm_callback_fixed('ch2pin');
      mask TypeOptions ch3pin: Not available - Do not use | A2 | B10
      mask Callback ch3pin: stm32f4_basicpwm_callback_fixed('ch3pin');
      mask TypeOptions ch4pin: Not available - Do not use | A3 | B11
      mask Callback ch4pin: stm32f4_basicpwm_callback_fixed('ch4pin');
      mask Callback sampletime: stm32f4_basicpwm_callback_fixed('sampletime');
      mask Callback sampletimestr: stm32f4_basicpwm_callback_fixed('sampletimestr');
      mask Callback blockid: stm32f4_basicpwm_callback_fixed('blockid');
      mask Callback enablecustomportlabel: stm32f4_basicpwm_callback_fixed('enablecustomportlabel')
      mask Display: text(0.95, 0.5, 'UC3M FIXED\nTimer: 2\nPolarity: Active High\nPeriod (sec): 0.0002\nTs (sec): -1','ver','middle','hor','right');port_label('input', 1,'CH3 (A2)')
  "Velocty wheel 1, analog in (Grey), PC4" : stm32f4_adc_lib/Regular ADC  Commented=on  adcmodule=1  outputdatatype=Double  prescaler=2  prescalerstr=ADC_Prescaler_Div2  chsamplingtime=Auto  chsamplingtimestr=ADC_SampleTime_480Cycles  read_an0=off  read_an1=off  read_an2=off  read_an3=off  read_an4=off  read_an5=off  read_an6=off  read_an7=off  read_an8=off  read_an9=off  read_an10=off  read_an11=off  read_an12=off  read_an13=off  read_an14=on  read_an15=off  read_an16=off  read_an17=off  read_an18=off  pinstr=GPIO_Pin_14  usedpinarray="[0  0  0  0  0  0  0  0  0  0  0  0  0  0  1  0  0  0  0]"  usedportidarray=[2]  usedpinidarray=[4]  usedpinidcount=1  sampletime=-1  blockid=motor1Veloctywheel1analoginGreyPC4  enablecustomportlabel=off  cinputportlabel=0  coutputportlabel=Out1, Out2
  wires:
  Ampere PWM/1 -> PWM Ampere motor 3 (white)/1
  "Direction Motor "/1 -> Direction Motor 3 (green)/1
  Enable Motor/1 -> Enable Motor 3(yellow)/1

== system CubeX_LQR_3D/LQR/K matrix (LQR) ==
  State : Inport
  Gain : Gain  Gain=-K_lqr_3D  Multiplication=Matrix(K*u)
  M : Outport
  wires:
  Gain/1 -> M/1
  State/1 -> Gain/1

== system CubeX_LQR_3D/LQR/Torque to Current ==
  M : Inport
  Gain1 : Gain  Gain=1/motor.kt
  iref : Outport
  wires:
  M/1 -> Gain1/1
  Gain1/1 -> iref/1

== system CubeX_LQR_3D/Read IMU/Accelometer Gyroscope I2C1 ==
  SlvAddr MPU9250 : Inport
  Constant : Constant  Value=true  OutDataTypeStr=boolean  SampleTime=Ts.IMU
  MPU9250 Init : Subsystem  Commented=on
  Read Accelometer and Gyroscope Data : Subsystem
  acc : Outport
  gyro : Outport  Port=2
  wires:
  SlvAddr MPU9250/1 -> Read Accelometer and Gyroscope Data/1(SlvAddr)
  Read Accelometer and Gyroscope Data/1(acc) -> acc/1
  Read Accelometer and Gyroscope Data/2(gyro) -> gyro/1
  Constant/1 -> Read Accelometer and Gyroscope Data/Enable

== system CubeX_LQR_3D/Read IMU/Accelometer Gyroscope I2C3 ==
  SlvAddr MPU9250 : Inport
  Constant : Constant  Value=true  OutDataTypeStr=boolean  SampleTime=Ts.IMU
  MPU9250 Init : Subsystem  Commented=on
  Read Accelometer and Gyroscope Data : Subsystem
  acc : Outport
  gyro : Outport  Port=2
  wires:
  SlvAddr MPU9250/1 -> Read Accelometer and Gyroscope Data/1(SlvAddr)
  Read Accelometer and Gyroscope Data/1(acc) -> acc/1
  Read Accelometer and Gyroscope Data/2(gyro) -> gyro/1
  Constant/1 -> Read Accelometer and Gyroscope Data/Enable

== system CubeX_LQR_3D/Read IMU/Converting raw data to SI units ==
  acc_raw : Inport
  gyro_raw : Inport  Port=2
  Raw sensor value to SI units Accelometer : Gain  Gain=1 / imu.a_scaling * g
  Raw sensor value to SI units Gyroscope : Gain  Gain=1 / imu.w_scaling * deg_
  acc : Outport
  gyro : Outport  Port=2
  wires:
  gyro_raw/1 -> Raw sensor value to SI units Gyroscope/1
  Raw sensor value to SI units Accelometer/1 -> acc/1
  Raw sensor value to SI units Gyroscope/1 -> gyro/1
  acc_raw/1 -> Raw sensor value to SI units Accelometer/1

== system CubeX_LQR_3D/Read IMU/Light LED 4 on board when calibration is done ==
  IO : Inport
  Led : stm32f4_io_lib/Digital Output  use_bitband=on  port=D  speed=100  porttype=Push Pull  porttypestr=PP  use_pin0=off  use_pin1=off  use_pin2=off  use_pin3=off  use_pin4=off  use_pin5=off  use_pin6=off  use_pin7=off  use_pin8=off  use_pin9=off  use_pin10=off  use_pin11=off  use_pin12=on  use_pin13=off  use_pin14=off  use_pin15=off  pinstr=GPIO_Pin_12  usedpinarray="[0  0  0  0  0  0  0  0  0  0  0  0  1  0  0  0]"  bitbandingstr="#define ReadIMULightLED4onboardwhencalibrationisdoneLed_D12 Peripheral_BB(GPIOD->ODR, 12)  /* Output pin */"  sampletime=Ts.IMU  sampletimestr=0.008  blockid=ReadIMULightLED4onboardwhencalibrationisdoneLed  enablecustomportlabel=off  globalinit=off  cinputportlabel=In1, In2  coutputportlabel=0
  wires:
  IO/1 -> Led/1

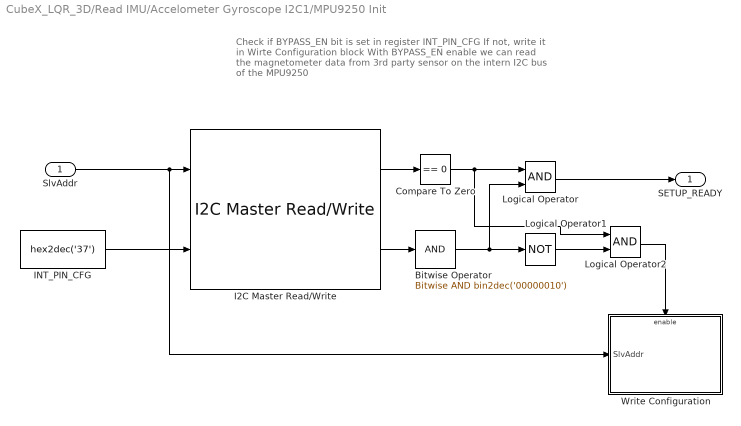
== system CubeX_LQR_3D/Read IMU/Accelometer Gyroscope I2C1/MPU9250 Init ==
  note: Check if BYPASS_EN bit is set in register INT_PIN_CFG
      | If not, write it in Wirte Configuration block
      |
      | With BYPASS_EN enable we can read the magnetometer data
      | from 3rd party sensor on the intern I2C bus of the MPU9250
  SlvAddr : Inport
  Bitwise Operator : simulink/Logic and Bit Operations/Bitwise Operator  logicop=AND  UseBitMask=on  BitMask=bin2dec('00000010')  BitMaskRealWorld=Stored Integer
  Compare To Zero : simulink/Logic and Bit Operations/Compare To Zero  relop===  OutDataTypeStr=boolean
  I2C Master Read/Write : stm32f4_i2c_lib/I2C Master Read//Write  configuration=Transaction  module=1  lastmodule=3  transfer=Blocking  dutycycle=TLow/THigh = 2  clkspeed=400  timeout=25  writecount=1  readcount=1  sdapin=C9  sclpin=A8  waitwritetime=0  forcestop=off  inputtypearray=[2 3 3]  outputtypearray=[2 3 3]  confstr="[\"C\",\"9\",\"A\",\"8\",\"1\",\"1\",\"6\",\"0\",\"I2C_DutyCycle_2\",\"0\",\"off\"]"  sampletime=-1  sampletimestr=0.008  blockid=ReadIMUAccelometerGyroscopeI2C1MPU9250InitI2CMasterReadWrite
  INT_PIN_CFG : Constant  Value=hex2dec('37')  OutDataTypeStr=uint8  SampleTime=-1
  Logical Operator : Logic  AllPortsSameDT=off  OutDataTypeStr=boolean
  Logical Operator1 : Logic  Operator=NOT  AllPortsSameDT=off  OutDataTypeStr=boolean
  Logical Operator2 : Logic  AllPortsSameDT=off  OutDataTypeStr=boolean
  Write Configuration : Subsystem
  SETUP_READY : Outport
  wires:
  I2C Master Read/Write/1 -> Compare To Zero/1
  INT_PIN_CFG/1 -> I2C Master Read/Write/2
  SlvAddr/1 -> Write Configuration/1(SlvAddr), I2C Master Read/Write/1
  Logical Operator/1 -> SETUP_READY/1
  Compare To Zero/1 -> Logical Operator2/1, Logical Operator/1
  Bitwise Operator/1 -> Logical Operator1/1, Logical Operator/2
  Logical Operator1/1 -> Logical Operator2/2
  Logical Operator2/1 -> Write Configuration/Enable
  I2C Master Read/Write/2 -> Bitwise Operator/1

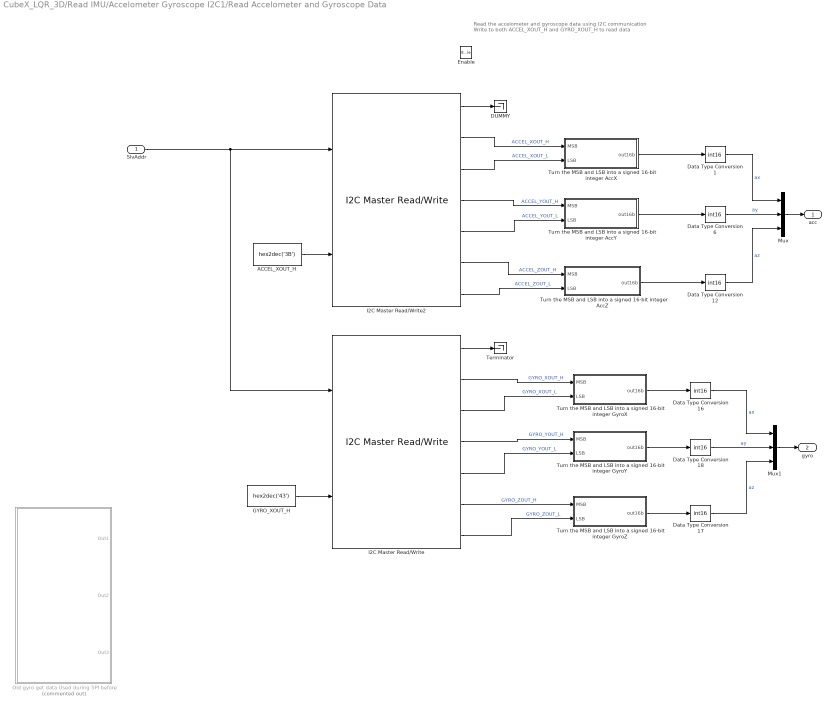
== system CubeX_LQR_3D/Read IMU/Accelometer Gyroscope I2C1/Read Accelometer and Gyroscope Data ==
  note: Read the accelometer and gyroscope data using I2C communication
      | Write to both ACCEL_XOUT_H and GYRO_XOUT_H to read data
  SlvAddr : Inport
  Enable : EnablePort
  ACCEL_XOUT_H : Constant  Value=hex2dec('3B')  OutDataTypeStr=uint8  SampleTime=-1
  DUMMY : Terminator
  Data Type Conversion{1,6,12,16..18} (6 alike) : DataTypeConversion  OutDataTypeStr=int16
  GYRO_XOUT_H : Constant  Value=hex2dec('43')  OutDataTypeStr=uint8  SampleTime=-1
  I2C Master Read/Write : stm32f4_i2c_lib/I2C Master Read//Write  configuration=Transaction  module=1  lastmodule=3  transfer=Blocking  dutycycle=TLow/THigh = 2  clkspeed=400  timeout=25  writecount=1  readcount=6  sdapin=C9  sclpin=A8  waitwritetime=0  forcestop=off  inputtypearray=[2 3 3]  outputtypearray=[7 3 3 3 3 3 3 3]  confstr="[\"C\",\"9\",\"A\",\"8\",\"1\",\"1\",\"6\",\"0\",\"I2C_DutyCycle_2\",\"0\",\"off\"]"  sampletime=Ts.IMU  sampletimestr=0.008  blockid=ReadIMUAccelometerGyroscopeI2C1ReadAccelometerandGyroscopeDataI2CMasterReadWrite
  I2C Master Read/Write2 : stm32f4_i2c_lib/I2C Master Read//Write  configuration=Transaction  module=1  lastmodule=3  transfer=Blocking  dutycycle=TLow/THigh = 2  clkspeed=400  timeout=25  writecount=1  readcount=6  sdapin=C9  sclpin=A8  waitwritetime=0  forcestop=off  inputtypearray=[2 3 3]  outputtypearray=[7 3 3 3 3 3 3 3]  confstr="[\"C\",\"9\",\"A\",\"8\",\"1\",\"1\",\"6\",\"0\",\"I2C_DutyCycle_2\",\"0\",\"off\"]"  sampletime=Ts.IMU  sampletimestr=0.008  blockid=ReadIMUAccelometerGyroscopeI2C1ReadAccelometerandGyroscopeDataI2CMasterReadWrite2
  Mux : Mux  Inputs=3
  Mux1 : Mux  Inputs=3
  Old gyro get data Used during SPI before : Subsystem  Commented=on
  Terminator : Terminator
  Turn the MSB and LSB into a signed 16-bit integer AccX : Subsystem
  Turn the MSB and LSB into a signed 16-bit integer AccY : Subsystem
  Turn the MSB and LSB into a signed 16-bit integer AccZ : Subsystem
  Turn the MSB and LSB into a signed 16-bit integer GyroX : Subsystem
  Turn the MSB and LSB into a signed 16-bit integer GyroY : Subsystem
  Turn the MSB and LSB into a signed 16-bit integer GyroZ : Subsystem
  acc : Outport
  gyro : Outport  Port=2
  wires:
  I2C Master Read/Write2/1 -> DUMMY/1
  Mux/1 -> acc/1
  Turn the MSB and LSB into a signed 16-bit integer AccX/1(out16b) -> Data Type Conversion1/1
  Turn the MSB and LSB into a signed 16-bit integer AccY/1(out16b) -> Data Type Conversion6/1
  Turn the MSB and LSB into a signed 16-bit integer AccZ/1(out16b) -> Data Type Conversion12/1
  Data Type Conversion1/1 -> Mux/1  "ax"
  Data Type Conversion6/1 -> Mux/2  "ay"
  Data Type Conversion12/1 -> Mux/3  "az"
  Mux1/1 -> gyro/1
  Turn the MSB and LSB into a signed 16-bit integer GyroX/1(out16b) -> Data Type Conversion16/1
  Turn the MSB and LSB into a signed 16-bit integer GyroY/1(out16b) -> Data Type Conversion18/1
  Turn the MSB and LSB into a signed 16-bit integer GyroZ/1(out16b) -> Data Type Conversion17/1
  Data Type Conversion16/1 -> Mux1/1  "ax"
  Data Type Conversion18/1 -> Mux1/2  "ay"
  Data Type Conversion17/1 -> Mux1/3  "az"
  GYRO_XOUT_H/1 -> I2C Master Read/Write/2
  ACCEL_XOUT_H/1 -> I2C Master Read/Write2/2
  SlvAddr/1 -> I2C Master Read/Write/1, I2C Master Read/Write2/1
  I2C Master Read/Write2/2 -> Turn the MSB and LSB into a signed 16-bit integer AccX/1(MSB)  "ACCEL_XOUT_H"
  I2C Master Read/Write2/3 -> Turn the MSB and LSB into a signed 16-bit integer AccX/2(LSB)  "ACCEL_XOUT_L"
  I2C Master Read/Write2/5 -> Turn the MSB and LSB into a signed 16-bit integer AccY/2(LSB)  "ACCEL_YOUT_L"
  I2C Master Read/Write2/4 -> Turn the MSB and LSB into a signed 16-bit integer AccY/1(MSB)  "ACCEL_YOUT_H"
  I2C Master Read/Write2/6 -> Turn the MSB and LSB into a signed 16-bit integer AccZ/1(MSB)  "ACCEL_ZOUT_H"
  I2C Master Read/Write2/7 -> Turn the MSB and LSB into a signed 16-bit integer AccZ/2(LSB)  "ACCEL_ZOUT_L"
  I2C Master Read/Write/2 -> Turn the MSB and LSB into a signed 16-bit integer GyroX/1(MSB)  "GYRO_XOUT_H"
  I2C Master Read/Write/3 -> Turn the MSB and LSB into a signed 16-bit integer GyroX/2(LSB)  "GYRO_XOUT_L"
  I2C Master Read/Write/4 -> Turn the MSB and LSB into a signed 16-bit integer GyroY/1(MSB)  "GYRO_YOUT_H"
  I2C Master Read/Write/5 -> Turn the MSB and LSB into a signed 16-bit integer GyroY/2(LSB)  "GYRO_YOUT_L"
  I2C Master Read/Write/6 -> Turn the MSB and LSB into a signed 16-bit integer GyroZ/1(MSB)  "GYRO_ZOUT_H"
  I2C Master Read/Write/7 -> Turn the MSB and LSB into a signed 16-bit integer GyroZ/2(LSB)  "GYRO_ZOUT_L"
  I2C Master Read/Write/1 -> Terminator/1

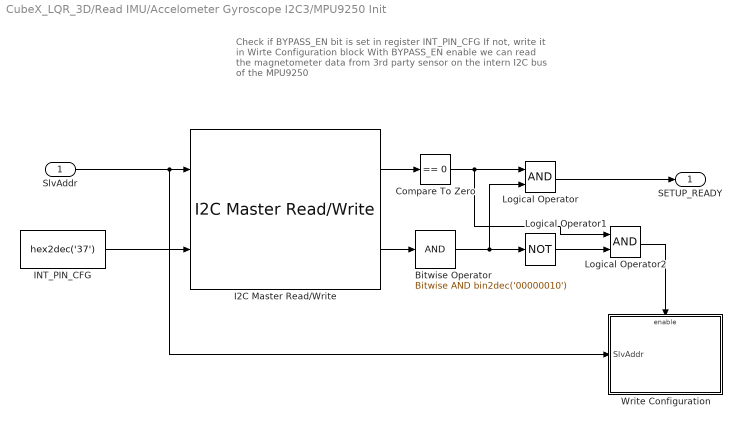
== system CubeX_LQR_3D/Read IMU/Accelometer Gyroscope I2C3/MPU9250 Init ==
  note: Check if BYPASS_EN bit is set in register INT_PIN_CFG
      | If not, write it in Wirte Configuration block
      |
      | With BYPASS_EN enable we can read the magnetometer data
      | from 3rd party sensor on the intern I2C bus of the MPU9250
  SlvAddr : Inport
  Bitwise Operator : simulink/Logic and Bit Operations/Bitwise Operator  logicop=AND  UseBitMask=on  BitMask=bin2dec('00000010')  BitMaskRealWorld=Stored Integer
  Compare To Zero : simulink/Logic and Bit Operations/Compare To Zero  relop===  OutDataTypeStr=boolean
  I2C Master Read/Write : stm32f4_i2c_lib/I2C Master Read//Write  configuration=Transaction  module=3  lastmodule=3  transfer=Blocking  dutycycle=TLow/THigh = 2  clkspeed=400  timeout=25  writecount=1  readcount=1  sdapin=C9  sclpin=A8  waitwritetime=0  forcestop=off  inputtypearray=[2 3 3]  outputtypearray=[2 3 3]  confstr="[\"C\",\"9\",\"A\",\"8\",\"1\",\"3\",\"4\",\"2\",\"I2C_DutyCycle_2\",\"0\",\"off\"]"  sampletime=-1  sampletimestr=0.008  blockid=ReadIMUAccelometerGyroscopeI2C3MPU9250InitI2CMasterReadWrite
  INT_PIN_CFG : Constant  Value=hex2dec('37')  OutDataTypeStr=uint8  SampleTime=-1
  Logical Operator : Logic  AllPortsSameDT=off  OutDataTypeStr=boolean
  Logical Operator1 : Logic  Operator=NOT  AllPortsSameDT=off  OutDataTypeStr=boolean
  Logical Operator2 : Logic  AllPortsSameDT=off  OutDataTypeStr=boolean
  Write Configuration : Subsystem
  SETUP_READY : Outport
  wires:
  I2C Master Read/Write/1 -> Compare To Zero/1
  INT_PIN_CFG/1 -> I2C Master Read/Write/2
  SlvAddr/1 -> Write Configuration/1(SlvAddr), I2C Master Read/Write/1
  Logical Operator/1 -> SETUP_READY/1
  Compare To Zero/1 -> Logical Operator2/1, Logical Operator/1
  Bitwise Operator/1 -> Logical Operator1/1, Logical Operator/2
  Logical Operator1/1 -> Logical Operator2/2
  Logical Operator2/1 -> Write Configuration/Enable
  I2C Master Read/Write/2 -> Bitwise Operator/1
